simulink model "SIMULINK_EX_III"  (R2021a)
settings: Solver=VariableStepAuto  StartTime=0.0  StopTime=10.0  RelTol=1e-3
settings Model: Creator=GHOST  LastModifiedBy=GHOST

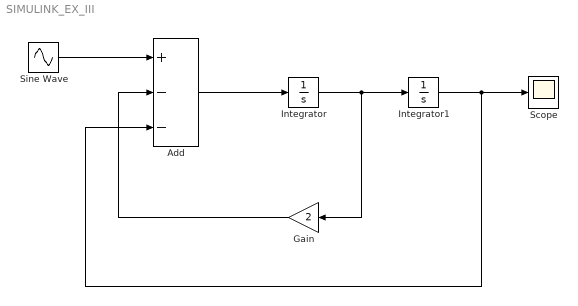
== system SIMULINK_EX_III ==
  Add : Sum  Inputs=+--
  Gain : Gain  Gain=2
  Integrator : Integrator
  Integrator1 : Integrator
  Scope : Scope
  Sine Wave : Sin  Frequency=2  SampleTime=0
  wires:
  Sine Wave/1 -> Add/1
  Add/1 -> Integrator/1
  Integrator/1 -> Gain/1, Integrator1/1
  Integrator1/1 -> Add/3, Scope/1
  Gain/1 -> Add/2
